simulink model "DFIG"  (R2019b)
settings: Solver=ode23t  StartTime=0.0  StopTime=60  RelTol=1e-3
undefined symbols (not defined in the file or in its folder): j
settings Model: Creator=ThinkPad  LastModifiedBy=pimou
settings DebuggingCC: UnconnectedInputMsg=none  UnconnectedOutputMsg=none  UnconnectedLineMsg=none
settings ModelReferenceCC: EnableRefExpFcnMdlSchedulingChecks=off
settings RTWCC: Description=Generic Real-Time Target

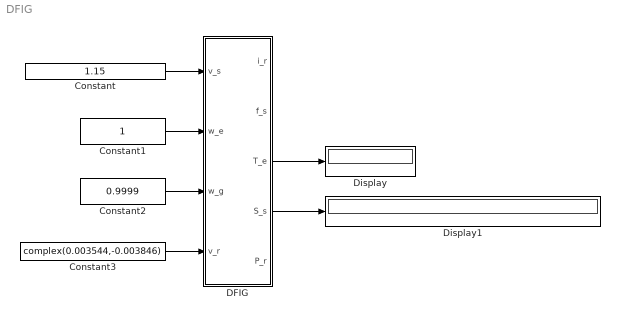
== system DFIG ==
  Constant : Constant  Value=1.15
  Constant1 : Constant
  Constant2 : Constant  Value=0.9999
  Constant3 : Constant  Value=complex(0.003544,-0.003846)
  DFIG : Subsystem  mask{R_s=4.62e-3, R_r=3.8e-3, L_m=1.99, L_s=118.18e-3}
  Display : Display
  Display1 : Display
  wires:
  DFIG/3(T_e) -> Display/1
  DFIG/4(S_s) -> Display1/1
  Constant/1 -> DFIG/1(v_s)
  Constant1/1 -> DFIG/2(w_e)
  Constant2/1 -> DFIG/3(w_g)
  Constant3/1 -> DFIG/4(v_r)

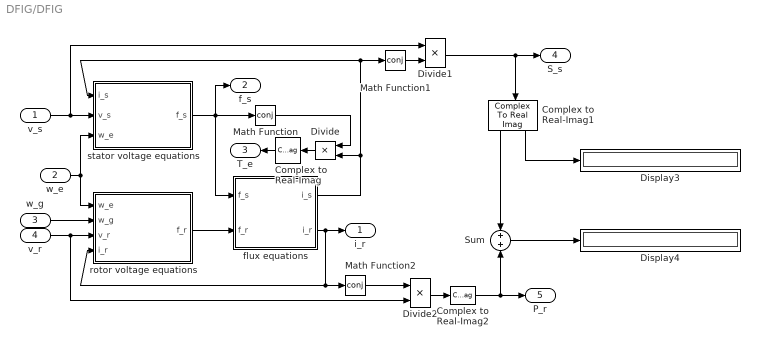
== system DFIG/DFIG ==
  v_s : Inport
  w_e : Inport  Port=2
  w_g : Inport  Port=3
  v_r : Inport  Port=4
  Complex to Real-Imag : ComplexToRealImag  Output=Imag
  Complex to Real-Imag1 : ComplexToRealImag
  Complex to Real-Imag2 : ComplexToRealImag  Output=Real
  Display3 : Display
  Display4 : Display
  Divide : Product  Inputs=**
  Divide1 : Product  Inputs=**
  Divide2 : Product  Inputs=**
  Math Function : Math  Operator=conj  SaturateOnIntegerOverflow=on
  Math Function1 : Math  Operator=conj  SaturateOnIntegerOverflow=on
  Math Function2 : Math  Operator=conj  SaturateOnIntegerOverflow=on
  Sum : Sum
  flux equations : Subsystem
  rotor voltage equations : Subsystem
  stator voltage equations : Subsystem
  i_r : Outport
  f_s : Outport  Port=2
  T_e : Outport  Port=3
  S_s : Outport  Port=4
  P_r : Outport  Port=5
  wires:
  Complex to Real-Imag2/1 -> Sum/2, P_r/1
  Math Function2/1 -> Divide2/1
  stator voltage equations/1(f_s) -> flux equations/1(f_s), f_s/1, Math Function/1
  Math Function/1 -> Divide/1
  Divide2/1 -> Complex to Real-Imag2/1
  Divide1/1 -> Complex to Real-Imag1/1, S_s/1
  Math Function1/1 -> Divide1/2
  Complex to Real-Imag/1 -> T_e/1
  Divide/1 -> Complex to Real-Imag/1
  rotor voltage equations/1(f_r) -> flux equations/2(f_r)
  flux equations/2(i_r) -> Math Function2/1, rotor voltage equations/4(i_r), i_r/1
  flux equations/1(i_s) -> Divide/2, stator voltage equations/1(i_s), Math Function1/1
  v_r/1 -> rotor voltage equations/3(v_r), Divide2/2
  w_e/1 -> rotor voltage equations/1(w_e), stator voltage equations/3(w_e)
  v_s/1 -> Divide1/1, stator voltage equations/2(v_s)
  w_g/1 -> rotor voltage equations/2(w_g)
  Sum/1 -> Display4/1
  Complex to Real-Imag1/1 -> Sum/1
  Complex to Real-Imag1/2 -> Display3/1

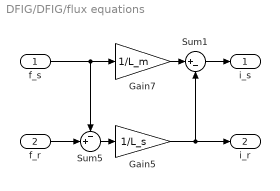
== system DFIG/DFIG/flux equations ==
  f_s : Inport
  f_r : Inport  Port=2
  Gain5 : Gain  Gain=1/L_s
  Gain7 : Gain  Gain=1/L_m
  Sum1 : Sum  Inputs=|+-
  Sum5 : Sum  Inputs=-+|
  i_s : Outport
  i_r : Outport  Port=2
  wires:
  Sum1/1 -> i_s/1
  Gain7/1 -> Sum1/1
  Sum5/1 -> Gain5/1
  f_r/1 -> Sum5/2
  Gain5/1 -> Sum1/2, i_r/1
  f_s/1 -> Sum5/1, Gain7/1

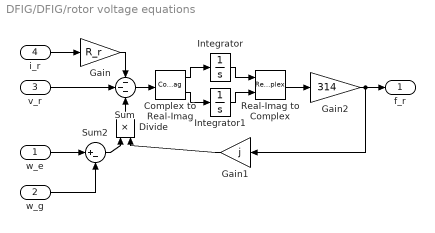
== system DFIG/DFIG/rotor voltage equations ==
  w_e : Inport
  w_g : Inport  Port=2
  v_r : Inport  Port=3
  i_r : Inport  Port=4
  Complex to Real-Imag : ComplexToRealImag
  Divide : Product  Inputs=**
  Gain : Gain  Gain=R_r
  Gain1 : Gain  Gain=j
  Gain2 : Gain  Gain=314
  Integrator : Integrator
  Integrator1 : Integrator
  Real-Imag to Complex : RealImagToComplex
  Sum : Sum  Inputs=---
  Sum2 : Sum  Inputs=|+-
  f_r : Outport
  wires:
  Gain2/1 -> Gain1/1, f_r/1
  Gain1/1 -> Divide/2
  Complex to Real-Imag/2 -> Integrator1/1
  Complex to Real-Imag/1 -> Integrator/1
  Sum/1 -> Complex to Real-Imag/1
  w_g/1 -> Sum2/2
  w_e/1 -> Sum2/1
  Gain/1 -> Sum/1
  v_r/1 -> Sum/2
  i_r/1 -> Gain/1
  Real-Imag to Complex/1 -> Gain2/1
  Sum2/1 -> Divide/1
  Divide/1 -> Sum/3
  Integrator1/1 -> Real-Imag to Complex/2
  Integrator/1 -> Real-Imag to Complex/1

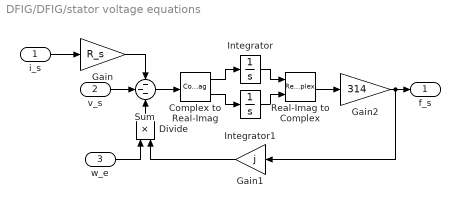
== system DFIG/DFIG/stator voltage equations ==
  i_s : Inport
  v_s : Inport  Port=2
  w_e : Inport  Port=3
  Complex to Real-Imag : ComplexToRealImag
  Divide : Product  Inputs=**
  Gain : Gain  Gain=R_s
  Gain1 : Gain  Gain=j
  Gain2 : Gain  Gain=314
  Integrator : Integrator
  Integrator1 : Integrator
  Real-Imag to Complex : RealImagToComplex
  Sum : Sum  Inputs=---
  f_s : Outport
  wires:
  Gain2/1 -> Gain1/1, f_s/1
  Gain1/1 -> Divide/2
  Complex to Real-Imag/2 -> Integrator1/1
  Complex to Real-Imag/1 -> Integrator/1
  Sum/1 -> Complex to Real-Imag/1
  v_s/1 -> Sum/2
  Gain/1 -> Sum/1
  i_s/1 -> Gain/1
  Real-Imag to Complex/1 -> Gain2/1
  w_e/1 -> Divide/1
  Divide/1 -> Sum/3
  Integrator1/1 -> Real-Imag to Complex/2
  Integrator/1 -> Real-Imag to Complex/1
